simulink model "GolfSwingZVCF"  (R2024b)
settings: Solver=VariableStepAuto  StartTime=0.0  StopTime=StopTime  MaxStep=0.001  RelTol=1e-3
PreLoadFcn:
  | cd(matlabdrive);
  | cd '2DModel';
PostLoadFcn:
  | %run SCRIPT_mdlWksGenerate.m;
  | mdlWks=get_param('GolfSwingZVCF','ModelWorkspace');
  | mdlWks.DataSource = 'MAT-File';
  | mdlWks.FileName = 'ModelInputs.mat';
  | mdlWks.reload;
model workspace: external: MAT-File ModelInputsZVCF.mat (data not in the file)
undefined symbols (not defined in the file): JointTorqueHip, JointTorqueLElbow, JointTorqueLScap, JointTorqueLShoulder, JointTorqueLWrist, JointTorqueRElbow, JointTorqueRScap, JointTorqueRShoulder, JointTorqueRWrist, JointTorqueTorso, X, Y, Z
libraries: nesl_utility x286, sm_lib x176, matrix_library x11, simulink_extras x2
(part 6 of 9)

== system GolfSwingZVCF/Club/Moment of Force Calculation/Convert to Local Moment ==
  LWMOFGlobal : Inport
  MPMOFGlobal : Inport  Port=2
  RWMOFGlobal : Inport  Port=3
  LeftHandMOFLocal : Product  Multiplication=Matrix(*)
  MidpointMOFLocal : Product  Multiplication=Matrix(*)
  RightHandMOFLocal : Product  Multiplication=Matrix(*)
  RotationTransformLeftHand : nesl_utility/PS-Simulink Converter  PhysicalDomain=network_engine_domain  SubClassName=ps_output  LeftPortType=input  RightPortType=output  PseudoPeriodic=off  Frequencies=[]  VectorFormat=1-D array  Unit=inherit  AffineConversion=off
  RotationTransformMidpoint : nesl_utility/PS-Simulink Converter  PhysicalDomain=network_engine_domain  SubClassName=ps_output  LeftPortType=input  RightPortType=output  PseudoPeriodic=off  Frequencies=[]  VectorFormat=1-D array  Unit=inherit  AffineConversion=off
  RotationTransformRightHand : nesl_utility/PS-Simulink Converter  PhysicalDomain=network_engine_domain  SubClassName=ps_output  LeftPortType=input  RightPortType=output  PseudoPeriodic=off  Frequencies=[]  VectorFormat=1-D array  Unit=inherit  AffineConversion=off
  Transform Sensor : sm_lib/Frames and Transforms/Transform Sensor  MeasurementFrame=World  RotationSequence=XYX  SenseAngle=off  SenseAxis=off  SenseQ=off  SenseR=on  SenseRotationSequence=off  SenseOmegaX=off  SenseOmegaY=off  SenseOmegaZ=off  SenseOmega=off  SenseQDot=off  SenseRDot=off  SenseRotationSequenceDot=off  SenseAlphaX=off  SenseAlphaY=off  SenseAlphaZ=off  SenseAlpha=off  SenseQDDot=off  SenseRDDot=off  SenseX=off  SenseY=off  SenseZ=off  SenseXYZ=off  SenseRad=off  SenseAzim=off  SenseDist=off  SenseInc=off  SenseXDot=off  SenseYDot=off  SenseZDot=off  SenseXYZDot=off  SenseRadDot=off  SenseAzimDot=off  SenseDistDot=off  SenseIncDot=off  SenseXDDot=off  SenseYDDot=off  SenseZDDot=off  SenseXYZDDot=off  SenseRadDDot=off  SenseAzimDDot=off  SenseDistDDot=off  SenseIncDDot=off
  Transform Sensor1 : sm_lib/Frames and Transforms/Transform Sensor  MeasurementFrame=World  RotationSequence=XYX  SenseAngle=off  SenseAxis=off  SenseQ=off  SenseR=on  SenseRotationSequence=off  SenseOmegaX=off  SenseOmegaY=off  SenseOmegaZ=off  SenseOmega=off  SenseQDot=off  SenseRDot=off  SenseRotationSequenceDot=off  SenseAlphaX=off  SenseAlphaY=off  SenseAlphaZ=off  SenseAlpha=off  SenseQDDot=off  SenseRDDot=off  SenseX=off  SenseY=off  SenseZ=off  SenseXYZ=off  SenseRad=off  SenseAzim=off  SenseDist=off  SenseInc=off  SenseXDot=off  SenseYDot=off  SenseZDot=off  SenseXYZDot=off  SenseRadDot=off  SenseAzimDot=off  SenseDistDot=off  SenseIncDot=off  SenseXDDot=off  SenseYDDot=off  SenseZDDot=off  SenseXYZDDot=off  SenseRadDDot=off  SenseAzimDDot=off  SenseDistDDot=off  SenseIncDDot=off
  Transform Sensor2 : sm_lib/Frames and Transforms/Transform Sensor  MeasurementFrame=World  RotationSequence=XYX  SenseAngle=off  SenseAxis=off  SenseQ=off  SenseR=on  SenseRotationSequence=off  SenseOmegaX=off  SenseOmegaY=off  SenseOmegaZ=off  SenseOmega=off  SenseQDot=off  SenseRDot=off  SenseRotationSequenceDot=off  SenseAlphaX=off  SenseAlphaY=off  SenseAlphaZ=off  SenseAlpha=off  SenseQDDot=off  SenseRDDot=off  SenseX=off  SenseY=off  SenseZ=off  SenseXYZ=off  SenseRad=off  SenseAzim=off  SenseDist=off  SenseInc=off  SenseXDot=off  SenseYDot=off  SenseZDot=off  SenseXYZDot=off  SenseRadDot=off  SenseAzimDot=off  SenseDistDot=off  SenseIncDot=off  SenseXDDot=off  SenseYDDot=off  SenseZDDot=off  SenseXYZDDot=off  SenseRadDDot=off  SenseAzimDDot=off  SenseDistDDot=off  SenseIncDDot=off
  World Frame : sm_lib/Frames and Transforms/World Frame
  LeftWrist : PMIOPort  Side=Left
  Midpoint : PMIOPort  Port=2  Side=Left
  RightWrist : PMIOPort  Port=3  Side=Left
  wires:
  RWMOFGlobal/1 -> RightHandMOFLocal/2
  MPMOFGlobal/1 -> MidpointMOFLocal/2
  RotationTransformLeftHand/1 -> LeftHandMOFLocal/1
  LWMOFGlobal/1 -> LeftHandMOFLocal/2
  RotationTransformMidpoint/1 -> MidpointMOFLocal/1
  RotationTransformRightHand/1 -> RightHandMOFLocal/1
  connections:
  World Frame/RConn1 -- Transform Sensor2/RConn1 -- Transform Sensor1/RConn1 -- Transform Sensor/RConn1
  RotationTransformLeftHand/LConn1 -- Transform Sensor/RConn2
  RotationTransformMidpoint/LConn1 -- Transform Sensor1/RConn2
  RotationTransformRightHand/LConn1 -- Transform Sensor2/RConn2
  Midpoint/RConn1 -- Transform Sensor1/LConn1
  LeftWrist/RConn1 -- Transform Sensor/LConn1
  RightWrist/RConn1 -- Transform Sensor2/LConn1

== system GolfSwingZVCF/Club/Moment of Force Calculation/Equivalent MP Couple ==
  LHMOFGlobal : Inport
  MPMOFGlobal : Inport  Port=2
  RHMOFGlobal : Inport  Port=3
  LWTorqueGlobal : Inport  Port=4
  RWTorqueGlobal : Inport  Port=5
  Convert Equivalent Midpoint Couple to Local Coordinates : Subsystem
  Convert Sum of Moments to Local Coordinates : Subsystem
  Equivalent Midhands Couple Global : Sum  Inputs=+-
  Sum of Moments Global : Sum  Inputs=++++
  MidpointConnection : PMIOPort  Side=Left
  wires:
  Sum of Moments Global/1 -> Convert Sum of Moments to Local Coordinates/1(SumofMomentsonClubGlobal), Equivalent Midhands Couple Global/1  "SumofMomentsonClubGlobal"
  LHMOFGlobal/1 -> Sum of Moments Global/1
  RWTorqueGlobal/1 -> Sum of Moments Global/4
  RHMOFGlobal/1 -> Sum of Moments Global/2
  MPMOFGlobal/1 -> Equivalent Midhands Couple Global/2
  LWTorqueGlobal/1 -> Sum of Moments Global/3
  Equivalent Midhands Couple Global/1 -> Convert Equivalent Midpoint Couple to Local Coordinates/1(EquivalentMidpointCoupleGlobal)  "EquivalentMidpointCoupleGlobal"
  connections:
  MidpointConnection/RConn1 -- Convert Sum of Moments to Local Coordinates/LConn1 -- Convert Equivalent Midpoint Couple to Local Coordinates/LConn1

== system GolfSwingZVCF/Club/Revolute Joint Shaft Models/12 Segment Shaft (1 Degree Prestress) ==
  Shaft Parameters : Subsystem
      settings: PortSchema="{\"entries\":[{\"content\":{\"sides\":[{\"content\":{\"connectorIds\":[\"Out13\"]},\"type\":\"ConnectorPlacement.EquallySpacedRectSide\",\"uuid\":\"090d18f5-fba2-4777-950b-42c4256e3ce5\"},{\"content\":{\"side\":\"RIGHT\"},\"type\":\"ConnectorPlacement.EquallySpacedRectSide\",\"uuid\":\"22324507-8879-4608-8b7a-b717aca1fc3d\"},{\"content\":{\"side\":\"TOP\"},\"type\":\"ConnectorPlacement.EquallySpacedRectSide\",\"uuid\":\"78aee44a-c65b-40dc-8adb-4dbd75f9d06e\"},{\"content\":{\"connectorIds\":[\"Out1\",\"Out2\",\"Out3\",\"Out4\",\"Out5\",\"Out6\",\"Out7\",\"Out8\",\"Out9\",\"Out10\",\"Out11\",\"Out12\"],\"side\":\"BOTTOM\"},\"type\":\"ConnectorPlacement.EquallySpacedRectSide\",\"uuid\":\"ed2cfdae-c9e7-4f47-afe1-727068d5ca73\"}]},\"type\":\"ConnectorPlacement.EquallySpacedConnector\",\"uuid\":\"620b5b82-0dc3-45b6-b9b3-642c5ae0b35c\"}],\"packageUris\":[\"http://schema.mathworks.com/mf0/Connector/R2020b\"],\"version\":\"1.0\"}"
  ShaftPhysicalConfig : Subsystem
      settings: PortSchema="{\"entries\":[{\"content\":{\"sides\":[{\"content\":{},\"type\":\"ConnectorPlacement.EquallySpacedRectSide\",\"uuid\":\"7709b5af-59ea-4c26-acaf-c61ffb72e436\"},{\"content\":{\"connectorIds\":[\"RConn1\",\"RConn2\",\"In1\",\"In2\",\"In3\",\"In4\",\"In5\",\"In6\",\"In7\",\"In8\",\"In9\",\"In10\",\"In11\",\"In12\",\"In13\"],\"side\":\"RIGHT\"},\"type\":\"ConnectorPlacement.EquallySpacedRectSide\",\"uuid\":\"b7f132e8-7068-4bdd-85c3-75504dc7b31d\"},{\"content\":{\"side\":\"TOP\"},\"type\":\"ConnectorPlacement.EquallySpacedRectSide\",\"uuid\":\"5befa0c7-aa08-4285-9a42-3adc09a962ba\"}]},\"type\":\"ConnectorPlacement.EquallySpacedConnector\",\"uuid\":\"383227f6-bb7d-45cc-90ad-5d8a4dfe3df4\"}],\"packageUris\":[\"http://schema.mathworks.com/mf0/Connector/R2020b\"],\"version\":\"1.0\"}"
  RH : PMIOPort  Side=Right
  Clubhead : PMIOPort  Port=2  Side=Right
  wires:
  Shaft Parameters/3(KStiff3) -> ShaftPhysicalConfig/4(KShaft3)
  Shaft Parameters/8(KStiff8) -> ShaftPhysicalConfig/9(KShaft8)
  Shaft Parameters/1(KStiff1) -> ShaftPhysicalConfig/2(KShaft1)
  Shaft Parameters/2(KStiff2) -> ShaftPhysicalConfig/3(KShaft2)
  Shaft Parameters/13(Kill) -> ShaftPhysicalConfig/1(Kill)
  Shaft Parameters/6(KStiff6) -> ShaftPhysicalConfig/7(KShaft6)
  Shaft Parameters/11(KStiff11) -> ShaftPhysicalConfig/12(KShaft11)
  Shaft Parameters/4(KStiff4) -> ShaftPhysicalConfig/5(KShaft4)
  Shaft Parameters/10(KStiff10) -> ShaftPhysicalConfig/11(KShaft10)
  Shaft Parameters/5(KStiff5) -> ShaftPhysicalConfig/6(KShaft5)
  Shaft Parameters/7(KStiff7) -> ShaftPhysicalConfig/8(KShaft7)
  Shaft Parameters/12(KDamp) -> ShaftPhysicalConfig/13(KDamp)
  Shaft Parameters/9(KStiff9) -> ShaftPhysicalConfig/10(KShaft9)
  connections:
  ShaftPhysicalConfig/RConn1 -- RH/RConn1
  Clubhead/RConn1 -- ShaftPhysicalConfig/RConn2

== system GolfSwingZVCF/Club/Revolute Joint Shaft Models/12 Segment Shaft (No Prestress)  ==
  Shaft Parameters : Subsystem
      settings: PortSchema="{\"entries\":[{\"content\":{\"sides\":[{\"content\":{\"connectorIds\":[\"Out13\"]},\"type\":\"ConnectorPlacement.EquallySpacedRectSide\",\"uuid\":\"090d18f5-fba2-4777-950b-42c4256e3ce5\"},{\"content\":{\"side\":\"RIGHT\"},\"type\":\"ConnectorPlacement.EquallySpacedRectSide\",\"uuid\":\"22324507-8879-4608-8b7a-b717aca1fc3d\"},{\"content\":{\"side\":\"TOP\"},\"type\":\"ConnectorPlacement.EquallySpacedRectSide\",\"uuid\":\"78aee44a-c65b-40dc-8adb-4dbd75f9d06e\"},{\"content\":{\"connectorIds\":[\"Out1\",\"Out2\",\"Out3\",\"Out4\",\"Out5\",\"Out6\",\"Out7\",\"Out8\",\"Out9\",\"Out10\",\"Out11\",\"Out12\"],\"side\":\"BOTTOM\"},\"type\":\"ConnectorPlacement.EquallySpacedRectSide\",\"uuid\":\"ed2cfdae-c9e7-4f47-afe1-727068d5ca73\"}]},\"type\":\"ConnectorPlacement.EquallySpacedConnector\",\"uuid\":\"620b5b82-0dc3-45b6-b9b3-642c5ae0b35c\"}],\"packageUris\":[\"http://schema.mathworks.com/mf0/Connector/R2020b\"],\"version\":\"1.0\"}"
  ShaftPhysicalConfig : Subsystem
      settings: PortSchema="{\"entries\":[{\"content\":{\"sides\":[{\"content\":{},\"type\":\"ConnectorPlacement.EquallySpacedRectSide\",\"uuid\":\"7709b5af-59ea-4c26-acaf-c61ffb72e436\"},{\"content\":{\"connectorIds\":[\"RConn1\",\"RConn2\",\"In1\",\"In2\",\"In3\",\"In4\",\"In5\",\"In6\",\"In7\",\"In8\",\"In9\",\"In10\",\"In11\",\"In12\",\"In13\"],\"side\":\"RIGHT\"},\"type\":\"ConnectorPlacement.EquallySpacedRectSide\",\"uuid\":\"b7f132e8-7068-4bdd-85c3-75504dc7b31d\"},{\"content\":{\"side\":\"TOP\"},\"type\":\"ConnectorPlacement.EquallySpacedRectSide\",\"uuid\":\"5befa0c7-aa08-4285-9a42-3adc09a962ba\"}]},\"type\":\"ConnectorPlacement.EquallySpacedConnector\",\"uuid\":\"383227f6-bb7d-45cc-90ad-5d8a4dfe3df4\"}],\"packageUris\":[\"http://schema.mathworks.com/mf0/Connector/R2020b\"],\"version\":\"1.0\"}"
  RH : PMIOPort  Side=Right
  Clubhead : PMIOPort  Port=2  Side=Right
  wires:
  Shaft Parameters/3(KStiff3) -> ShaftPhysicalConfig/4(KShaft3)
  Shaft Parameters/8(KStiff8) -> ShaftPhysicalConfig/9(KShaft8)
  Shaft Parameters/1(KStiff1) -> ShaftPhysicalConfig/2(KShaft1)
  Shaft Parameters/2(KStiff2) -> ShaftPhysicalConfig/3(KShaft2)
  Shaft Parameters/13(Kill) -> ShaftPhysicalConfig/1(Kill)
  Shaft Parameters/6(KStiff6) -> ShaftPhysicalConfig/7(KShaft6)
  Shaft Parameters/11(KStiff11) -> ShaftPhysicalConfig/12(KShaft11)
  Shaft Parameters/4(KStiff4) -> ShaftPhysicalConfig/5(KShaft4)
  Shaft Parameters/10(KStiff10) -> ShaftPhysicalConfig/11(KShaft10)
  Shaft Parameters/5(KStiff5) -> ShaftPhysicalConfig/6(KShaft5)
  Shaft Parameters/7(KStiff7) -> ShaftPhysicalConfig/8(KShaft7)
  Shaft Parameters/12(KDamp) -> ShaftPhysicalConfig/13(KDamp)
  Shaft Parameters/9(KStiff9) -> ShaftPhysicalConfig/10(KShaft9)
  connections:
  ShaftPhysicalConfig/RConn1 -- RH/RConn1
  Clubhead/RConn1 -- ShaftPhysicalConfig/RConn2

== system GolfSwingZVCF/Club/Zero Mass Reference Shaft/CHSCalculation ==
  In2 : Inport
  In3 : Inport  Port=2
  In1 : Inport  Port=3
  Add : Sum  Inputs=+++
  Math Function : Math  Operator=square
  Math Function1 : Math  Operator=square
  Math Function2 : Math  Operator=square
  Sqrt : Sqrt
  Out1 : Outport
  wires:
  Math Function2/1 -> Add/3
  In1/1 -> Math Function/1
  In2/1 -> Math Function1/1
  Math Function/1 -> Add/1
  Add/1 -> Sqrt/1
  In3/1 -> Math Function2/1
  Sqrt/1 -> Out1/1
  Math Function1/1 -> Add/2

== system GolfSwingZVCF/Club/Zero Mass Reference Shaft/ShaftPhysicalConfig ==
  GhostShaft : sm_lib/Body Elements/Cylindrical Solid  CylinderRadius=0.01  CylinderRadiusUnits=m  CylinderLength=1  CylinderLengthUnits=m  ExportEntireGeometry=off  InertiaType=CalculateFromGeometry  BasedOnType=Mass  Density=500  DensityUnits=kg/m^3  Mass=0  MassUnits=kg  CenterOfMass=[0 0 0]  CenterOfMassUnits=m  MomentsOfInertia=[1 1 1]  MomentsOfInertiaUnits=kg*m^2  ProductsOfInertia=[0 0 0]  ProductsOfInertiaUnits=kg*m^2  GraphicType=FromGeometry  MarkerShape=Sphere  MarkerSize=10  GraphicVisPropType=SimpleVisualProperties  GraphicDiffuseColor=[0.2 0.2 1.0]  GraphicOpacity=1.0  GraphicSpecularColor=[0.5 0.5 0.5 1.0]  GraphicAmbientColor=[0.15 0.15 0.15 1.0]  GraphicEmissiveColor=[0.0 0.0 0.0 1.0]  GraphicShininess=75  DoExposeReferenceFrame=off  SerializedFrames=<Frames><Frame><Id>Frame1</Id><Value><Name>RHGripTOS</Name><Origin><Source>GeometricFeature</Source><FeatureName>top curve</FeatureName></Origin><PrimaryAxis><DefinedDirection>-X</DefinedDirection><Source>ReferenceFrame</Source><SourceDirection>+Z</SourceDirection><FeatureName></FeatureName></PrimaryAxis><SecondaryAxis><DefinedDirection>+Y</DefinedDirection><Source>ReferenceFrame</Source><SourceDirection>+X</SourceDirection><FeatureName></FeatureName></SecondaryAxis></Value></Frame><Frame><Id>Frame2</Id><Value><Name>GhostClubhead</Name><Origin><Source>GeometricFeature</Source><FeatureName>bottom curve</FeatureName></Origin><PrimaryAxis><DefinedDirection>+Z</DefinedDirection><Source>ReferenceFrame</Source><SourceDirection>+Z</SourceDirection><FeatureName></FeatureName></PrimaryAxis><SecondaryAxis><DefinedDirection>+X</DefinedDirection><Source>ReferenceFrame</Source><SourceDirection>+X</SourceDirection><FeatureName></FeatureName></SecondaryAxis></Value></Frame></Frames>
  PS-Simulink Converter14 : nesl_utility/PS-Simulink Converter  PhysicalDomain=network_engine_domain  SubClassName=ps_output  LeftPortType=input  RightPortType=output  PseudoPeriodic=off  Frequencies=[]  VectorFormat=inherit  Unit=inherit  AffineConversion=off
  RH : PMIOPort  Side=Right
  RH1 : PMIOPort  Port=2  Side=Right
  connections:
  GhostShaft/LConn1 -- RH/RConn1
  RH1/RConn1 -- GhostShaft/RConn1

== system GolfSwingZVCF/Club/Moment of Force Calculation/Equivalent MP Couple/Convert Equivalent Midpoint Couple to Local Coordinates ==
  EquivalentMidpointCoupleGlobal : Inport
  Equivalent Midpoint Couple Local : Product  Multiplication=Matrix(*)
  RotationTransformMidpoint : nesl_utility/PS-Simulink Converter  PhysicalDomain=network_engine_domain  SubClassName=ps_output  LeftPortType=input  RightPortType=output  PseudoPeriodic=off  Frequencies=[]  VectorFormat=1-D array  Unit=inherit  AffineConversion=off
  Transform Sensor1 : sm_lib/Frames and Transforms/Transform Sensor  MeasurementFrame=World  RotationSequence=XYX  SenseAngle=off  SenseAxis=off  SenseQ=off  SenseR=on  SenseRotationSequence=off  SenseOmegaX=off  SenseOmegaY=off  SenseOmegaZ=off  SenseOmega=off  SenseQDot=off  SenseRDot=off  SenseRotationSequenceDot=off  SenseAlphaX=off  SenseAlphaY=off  SenseAlphaZ=off  SenseAlpha=off  SenseQDDot=off  SenseRDDot=off  SenseX=off  SenseY=off  SenseZ=off  SenseXYZ=off  SenseRad=off  SenseAzim=off  SenseDist=off  SenseInc=off  SenseXDot=off  SenseYDot=off  SenseZDot=off  SenseXYZDot=off  SenseRadDot=off  SenseAzimDot=off  SenseDistDot=off  SenseIncDot=off  SenseXDDot=off  SenseYDDot=off  SenseZDDot=off  SenseXYZDDot=off  SenseRadDDot=off  SenseAzimDDot=off  SenseDistDDot=off  SenseIncDDot=off
  World Frame : sm_lib/Frames and Transforms/World Frame
  MidpointConnection : PMIOPort  Side=Left
  wires:
  EquivalentMidpointCoupleGlobal/1 -> Equivalent Midpoint Couple Local/2
  RotationTransformMidpoint/1 -> Equivalent Midpoint Couple Local/1
  connections:
  RotationTransformMidpoint/LConn1 -- Transform Sensor1/RConn2
  MidpointConnection/RConn1 -- Transform Sensor1/LConn1
  World Frame/RConn1 -- Transform Sensor1/RConn1

== system GolfSwingZVCF/Club/Moment of Force Calculation/Equivalent MP Couple/Convert Sum of Moments to Local Coordinates ==
  SumofMomentsonClubGlobal : Inport
  RotationTransformMidpoint1 : nesl_utility/PS-Simulink Converter  PhysicalDomain=network_engine_domain  SubClassName=ps_output  LeftPortType=input  RightPortType=output  PseudoPeriodic=off  Frequencies=[]  VectorFormat=1-D array  Unit=inherit  AffineConversion=off
  SumofMomentsonClubLocal : Product  Multiplication=Matrix(*)
  Transform Sensor2 : sm_lib/Frames and Transforms/Transform Sensor  MeasurementFrame=World  RotationSequence=XYX  SenseAngle=off  SenseAxis=off  SenseQ=off  SenseR=on  SenseRotationSequence=off  SenseOmegaX=off  SenseOmegaY=off  SenseOmegaZ=off  SenseOmega=off  SenseQDot=off  SenseRDot=off  SenseRotationSequenceDot=off  SenseAlphaX=off  SenseAlphaY=off  SenseAlphaZ=off  SenseAlpha=off  SenseQDDot=off  SenseRDDot=off  SenseX=off  SenseY=off  SenseZ=off  SenseXYZ=off  SenseRad=off  SenseAzim=off  SenseDist=off  SenseInc=off  SenseXDot=off  SenseYDot=off  SenseZDot=off  SenseXYZDot=off  SenseRadDot=off  SenseAzimDot=off  SenseDistDot=off  SenseIncDot=off  SenseXDDot=off  SenseYDDot=off  SenseZDDot=off  SenseXYZDDot=off  SenseRadDDot=off  SenseAzimDDot=off  SenseDistDDot=off  SenseIncDDot=off
  World Frame1 : sm_lib/Frames and Transforms/World Frame
  Midpoint : PMIOPort  Side=Left
  wires:
  RotationTransformMidpoint1/1 -> SumofMomentsonClubLocal/1
  SumofMomentsonClubGlobal/1 -> SumofMomentsonClubLocal/2
  connections:
  RotationTransformMidpoint1/LConn1 -- Transform Sensor2/RConn2
  World Frame1/RConn1 -- Transform Sensor2/RConn1
  Midpoint/RConn1 -- Transform Sensor2/LConn1

== system GolfSwingZVCF/Club/Revolute Joint Shaft Models/12 Segment Shaft (1 Degree Prestress)/Shaft Parameters ==
  Constant : Constant  Value=2000
  Constant1 : Constant  Value=1200
  Constant2 : Constant  Value=200
  Constant3 : Constant  Value=2.865
  Dampener Gain : Constant
  Product{,1..3} (4 alike) : Product
  Step : Step  Before=1  After=0  SampleTime=0
  Stiffness Gain : Constant
  KStiff1 : Outport
  KStiff2 : Outport  Port=2
  KStiff3 : Outport  Port=3
  KStiff4 : Outport  Port=4
  KStiff5 : Outport  Port=5
  KStiff6 : Outport  Port=6
  KStiff7 : Outport  Port=7
  KStiff8 : Outport  Port=8
  KStiff9 : Outport  Port=9
  KStiff10 : Outport  Port=10
  KStiff11 : Outport  Port=11
  KDamp : Outport  Port=12
  Kill : Outport  Port=13
  wires:
  Step/1 -> Kill/1
  Constant2/1 -> Product2/2
  Constant1/1 -> Product1/2
  Constant/1 -> Product/2
  Stiffness Gain/1 -> Product2/1, Product1/1, Product/1
  Dampener Gain/1 -> Product3/1
  Constant3/1 -> Product3/2
  Product/1 -> KStiff3/1, KStiff2/1, KStiff1/1
  Product1/1 -> KStiff8/1, KStiff7/1, KStiff6/1, KStiff5/1, KStiff4/1
  Product2/1 -> KStiff9/1, KStiff11/1, KStiff10/1
  Product3/1 -> KDamp/1
